simulink model "msm_pi"  (R2021b)
settings: Solver=daessc  StartTime=0.0  StopTime=simlength  MaxStep=Tc  RelTol=1e-3
values from neighbouring files (symbols this model uses):
  A = [-(b+b_theta)/J1 b_theta/J1 -1/J1; b_theta/J2 -(b+b_theta)/J2 1/J2;     k_theta -k_theta 0]    [msm_init.m]
  Ale = [-(b+b_theta)/J1 b_theta/J1 -1/J1 0;         b_theta/J2 -(b+b_theta)/J2 1/J2 1/J2;        k_theta -k_theta 0 0 ... (first row only)    [msm_init.m]
  B = [1/J1 0 0]'    [msm_init.m]
  Ble = [1/J1 0 0 0]'    [msm_init.m]
  C = [1 0 0]    [msm_init.m]
  Cle = [1 0 0 0]    [msm_init.m]
  load_torque = 10    [msm_init.m]
  simlength = 20    [msm_init.m]
  Tc = Ts    (= 0.0001)    [msm_init.m]
undefined symbols (not defined in the file or in its folder): ki1, ki2, kp1, kp2, Ks, L, Lle
libraries: nesl_utility x22, fl_lib x12, mass_spring_mass_lib x4
settings Model: Creator=dbagn  LastModifiedBy=dbagn
settings SolverCC: AlgebraicLoopSolver=TrustRegion
settings DataIOCC: ReturnWorkspaceOutputs=off
settings DebuggingCC: SFMachineParentedDataDiag=warning

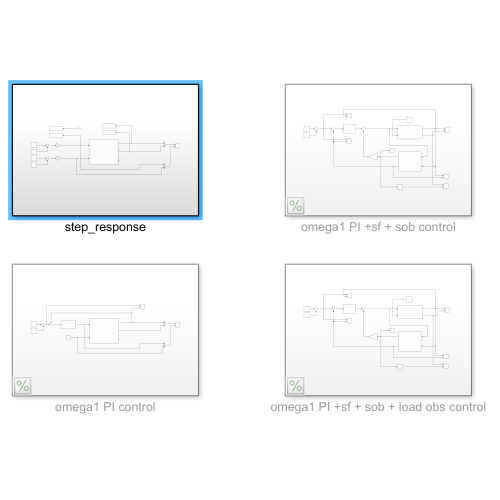
[thumbnail: Simulink's stored preview of the top-level diagram]
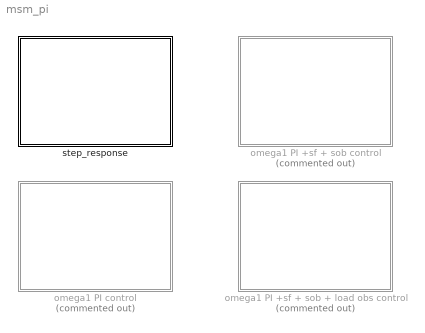
== system msm_pi ==
  omega1 PI +sf + sob + load obs control : Subsystem  Commented=on
  omega1 PI +sf + sob control : Subsystem  Commented=on
  omega1 PI control : Subsystem  Commented=on
  step_response : Subsystem

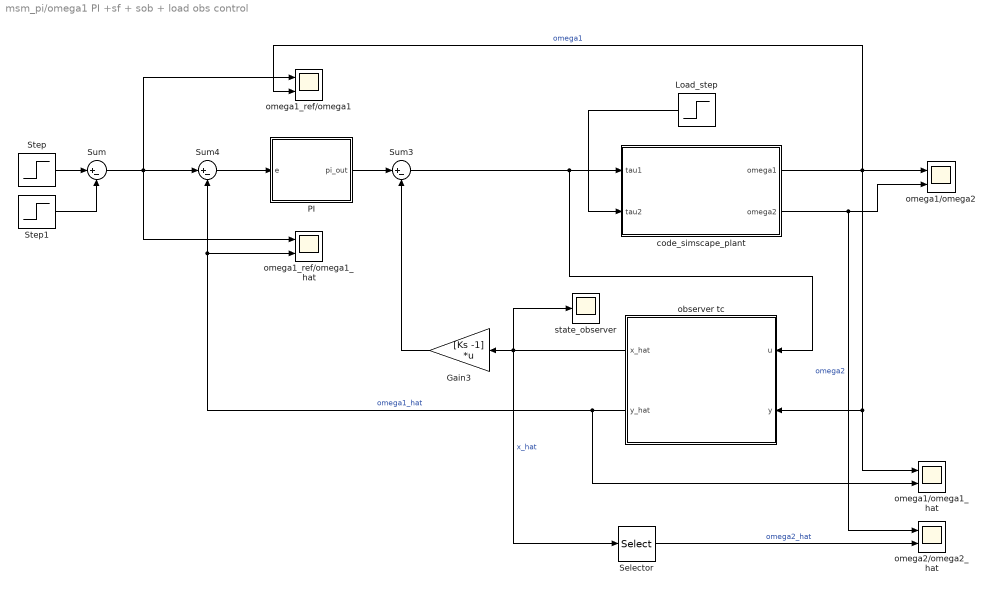
== system msm_pi/omega1 PI +sf + sob + load obs control ==
  Gain3 : Gain  Gain=[Ks -1]  Multiplication=Matrix(K*u)
  Load_step : Step  Time=16  After=load_torque  SampleTime=0
  PI : Subsystem
  Selector : Selector  InputPortWidth=4  IndexOptions=Index vector (dialog)  Indices=2  OutputSizes=1
  Step : Step  Time=0.2  SampleTime=0
  Step1 : Step  Time=8  SampleTime=0
  Sum : Sum  Inputs=|+-
  Sum3 : Sum  Inputs=|+-
  Sum4 : Sum  Inputs=|+-
  "code_simscape_plant " : Subsystem
  observer tc : Subsystem
  omega1/omega1_hat : Scope  NumInputPorts=2
  omega1/omega2 : Scope  NumInputPorts=2
  omega1_ref/omega1 : Scope  NumInputPorts=2
  omega1_ref/omega1_hat : Scope  NumInputPorts=2
  omega2/omega2_hat : Scope  NumInputPorts=2
  state_observer : Scope
  wires:
  PI/1(pi_out) -> Sum3/1
  "code_simscape_plant "/1(omega1) -> observer tc/2(y), omega1/omega1_hat/1, omega1/omega2/1, omega1_ref/omega1/2  "omega1"
  Sum4/1 -> PI/1(e)
  Load_step/1 -> "code_simscape_plant "/2(tau2)
  Gain3/1 -> Sum3/2
  "code_simscape_plant "/2(omega2) -> omega1/omega2/2, omega2/omega2_hat/1  "omega2"
  Selector/1 -> omega2/omega2_hat/2  "omega2_hat"
  observer tc/2(y_hat) -> omega1/omega1_hat/2, Sum4/2, omega1_ref/omega1_hat/2  "omega1_hat"
  observer tc/1(x_hat) -> Gain3/1, state_observer/1, Selector/1  "x_hat"
  Sum3/1 -> observer tc/1(u), "code_simscape_plant "/1(tau1)
  Step1/1 -> Sum/2
  Step/1 -> Sum/1
  Sum/1 -> omega1_ref/omega1_hat/1, Sum4/1, omega1_ref/omega1/1

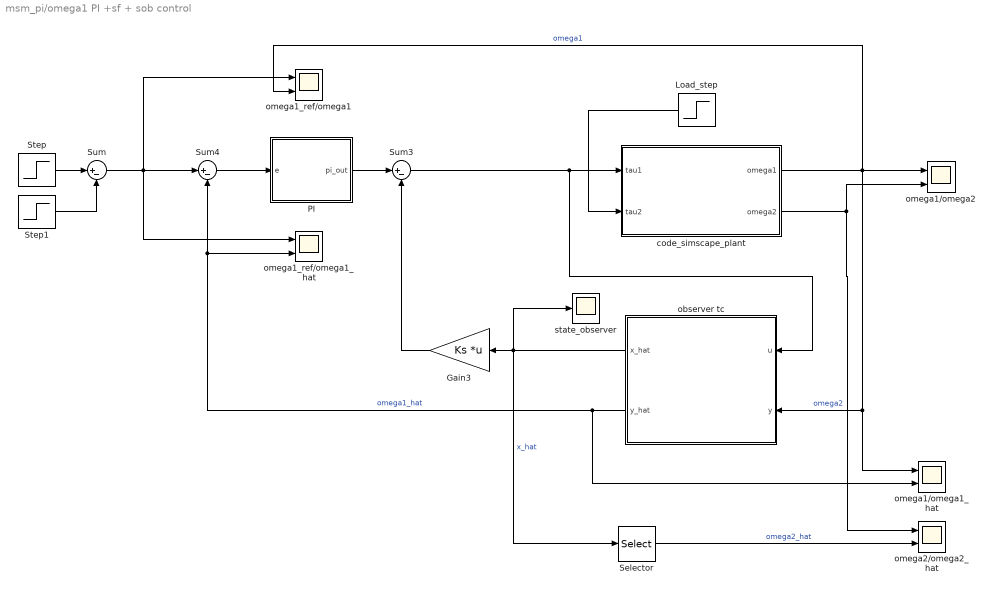
== system msm_pi/omega1 PI +sf + sob control ==
  Gain3 : Gain  Gain=Ks  Multiplication=Matrix(K*u)
  Load_step : Step  Time=16  After=load_torque  SampleTime=0
  PI : Subsystem
  Selector : Selector  InputPortWidth=3  IndexOptions=Index vector (dialog)  Indices=2  OutputSizes=1
  Step : Step  Time=0.2  SampleTime=0
  Step1 : Step  Time=8  SampleTime=0
  Sum : Sum  Inputs=|+-
  Sum3 : Sum  Inputs=|+-
  Sum4 : Sum  Inputs=|+-
  "code_simscape_plant " : Subsystem
  observer tc : Subsystem
  omega1/omega1_hat : Scope  NumInputPorts=2
  omega1/omega2 : Scope  NumInputPorts=2
  omega1_ref/omega1 : Scope  NumInputPorts=2
  omega1_ref/omega1_hat : Scope  NumInputPorts=2
  omega2/omega2_hat : Scope  NumInputPorts=2
  state_observer : Scope
  wires:
  Sum/1 -> omega1_ref/omega1/1, Sum4/1, omega1_ref/omega1_hat/1
  Step/1 -> Sum/1
  Step1/1 -> Sum/2
  Sum3/1 -> "code_simscape_plant "/1(tau1), observer tc/1(u)
  observer tc/1(x_hat) -> Selector/1, state_observer/1, Gain3/1  "x_hat"
  observer tc/2(y_hat) -> omega1_ref/omega1_hat/2, Sum4/2, omega1/omega1_hat/2  "omega1_hat"
  Selector/1 -> omega2/omega2_hat/2  "omega2_hat"
  "code_simscape_plant "/2(omega2) -> omega2/omega2_hat/1, omega1/omega2/2  "omega2"
  Gain3/1 -> Sum3/2
  Load_step/1 -> "code_simscape_plant "/2(tau2)
  Sum4/1 -> PI/1(e)
  "code_simscape_plant "/1(omega1) -> omega1_ref/omega1/2, omega1/omega2/1, omega1/omega1_hat/1, observer tc/2(y)  "omega1"
  PI/1(pi_out) -> Sum3/1

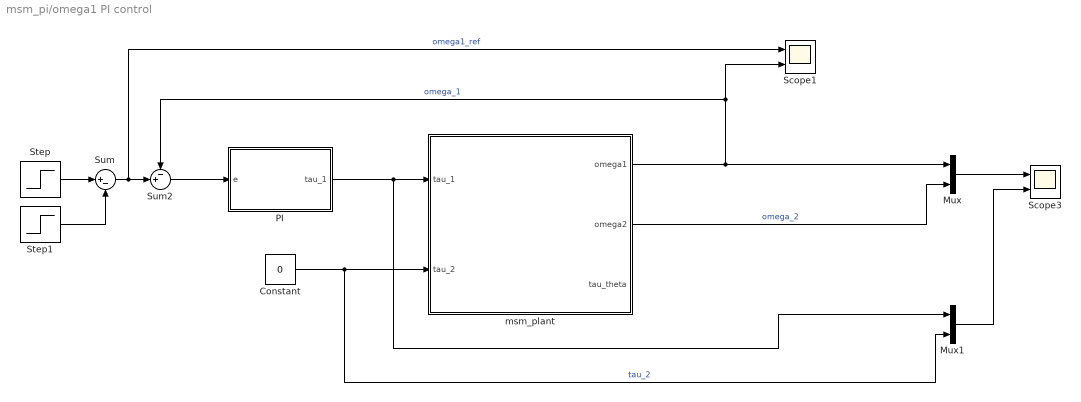
== system msm_pi/omega1 PI control ==
  Constant : Constant  Value=0
  Mux : Mux  Inputs=2
  Mux1 : Mux  Inputs=2
  PI : Subsystem
  Scope1 : Scope  NumInputPorts=2
  Scope3 : Scope  NumInputPorts=2
  Step : Step  Time=0.2  SampleTime=0
  Step1 : Step  Time=simlength/2  SampleTime=0
  Sum : Sum  Inputs=|+-
  Sum2 : Sum  Inputs=-+|
  msm_plant : Subsystem
  wires:
  Mux/1 -> Scope3/1
  Mux1/1 -> Scope3/2
  Step1/1 -> Sum/2
  Step/1 -> Sum/1
  msm_plant/2(omega2) -> Mux/2  "omega_2"
  msm_plant/1(omega1) -> Sum2/1, Scope1/2, Mux/1  "omega_1"
  Constant/1 -> msm_plant/2(tau_2), Mux1/2  "tau_2"
  Sum/1 -> Scope1/1, Sum2/2  "omega1_ref"
  PI/1(tau_1) -> Mux1/1, msm_plant/1(tau_1)
  Sum2/1 -> PI/1(e)

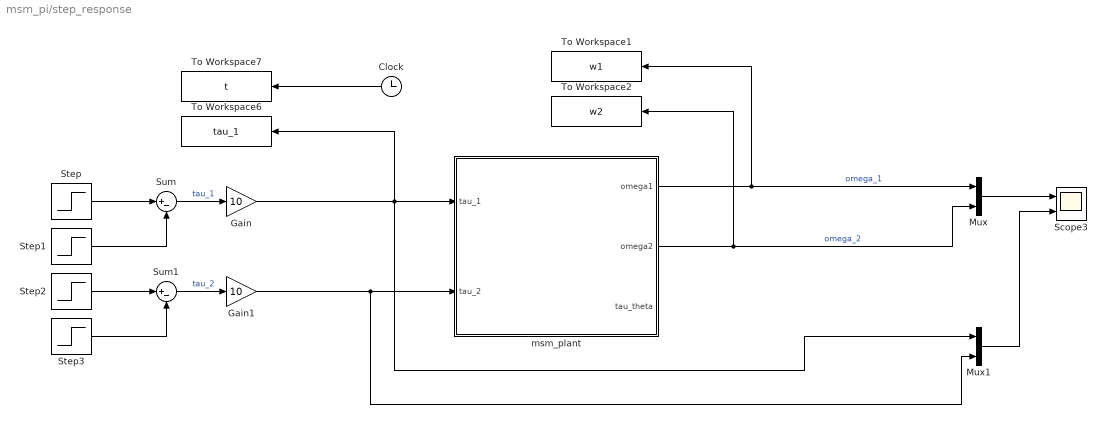
== system msm_pi/step_response ==
  Clock : Clock
  Gain : Gain  Gain=10
  Gain1 : Gain  Gain=10
  Mux : Mux  Inputs=2
  Mux1 : Mux  Inputs=2
  Scope3 : Scope  NumInputPorts=2
  Step : Step  Time=0.2  SampleTime=0
  Step1 : Step  Time=0.25  SampleTime=0
  Step2 : Step  Time=0.2+simlength/2  SampleTime=0
  Step3 : Step  Time=0.25+simlength/2  SampleTime=0
  Sum : Sum  Inputs=|+-
  Sum1 : Sum  Inputs=|+-
  To Workspace1 : ToWorkspace  VariableName=w1  SampleTime=Tc
      settings: MaxDataPoints=Nc
  To Workspace2 : ToWorkspace  VariableName=w2  SampleTime=Tc
      settings: MaxDataPoints=Nc
  To Workspace6 : ToWorkspace  VariableName=tau_1  SampleTime=Tc
      settings: MaxDataPoints=Nc
  To Workspace7 : ToWorkspace  VariableName=t  SampleTime=Tc
      settings: MaxDataPoints=Nc
  msm_plant : Subsystem
  wires:
  Step2/1 -> Sum1/1
  Sum1/1 -> Gain1/1  "tau_2"
  Step3/1 -> Sum1/2
  msm_plant/1(omega1) -> Mux/1, To Workspace1/1  "omega_1"
  Clock/1 -> To Workspace7/1
  msm_plant/2(omega2) -> Mux/2, To Workspace2/1  "omega_2"
  Sum/1 -> Gain/1  "tau_1"
  Step/1 -> Sum/1
  Step1/1 -> Sum/2
  Mux1/1 -> Scope3/2
  Mux/1 -> Scope3/1
  Gain/1 -> To Workspace6/1, Mux1/1, msm_plant/1(tau_1)
  Gain1/1 -> Mux1/2, msm_plant/2(tau_2)

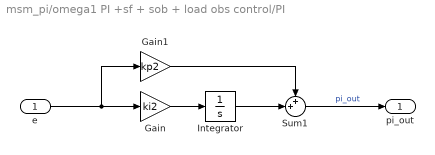
== system msm_pi/omega1 PI +sf + sob + load obs control/PI ==
  e : Inport
  Gain : Gain  Gain=ki2
  Gain1 : Gain  Gain=kp2
  Integrator : Integrator
  Sum1 : Sum  Inputs=++|
  pi_out : Outport
  wires:
  Sum1/1 -> pi_out/1  "pi_out"
  Gain1/1 -> Sum1/1
  Integrator/1 -> Sum1/2
  Gain/1 -> Integrator/1
  e/1 -> Gain1/1, Gain/1

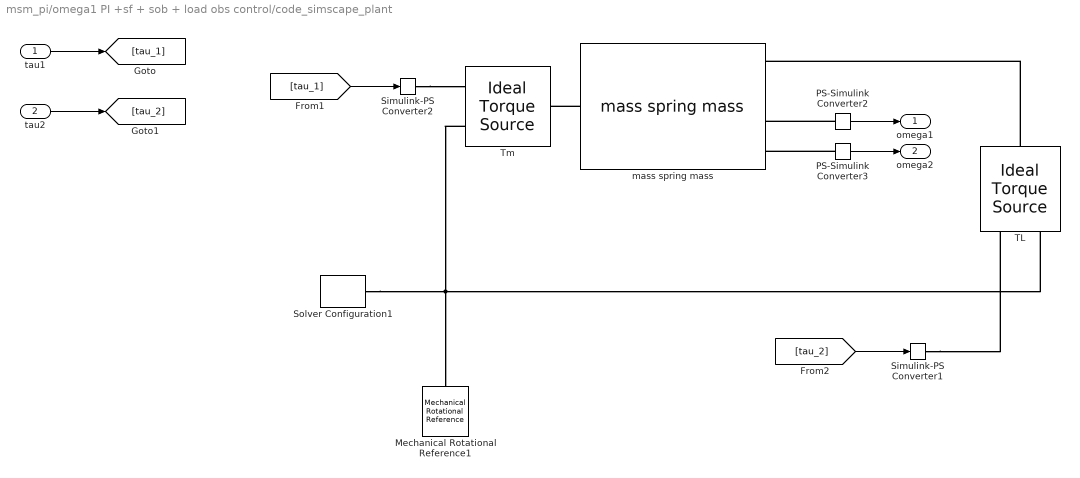
== system msm_pi/omega1 PI +sf + sob + load obs control/code_simscape_plant  ==
  tau1 : Inport
  tau2 : Inport  Port=2
  Mechanical Rotational Reference1 : fl_lib/Mechanical/Rotational Elements/Mechanical Rotational Reference
  PS-Simulink Converter2 : nesl_utility/PS-Simulink Converter  PhysicalDomain=network_engine_domain  SubClassName=ps_output  LeftPortType=input  RightPortType=output  PseudoPeriodic=off  Frequencies=[]  Unit=1  AffineConversion=off
      settings: SourceProductBaseCode=PW,SS
  PS-Simulink Converter3 : nesl_utility/PS-Simulink Converter  PhysicalDomain=network_engine_domain  SubClassName=ps_output  LeftPortType=input  RightPortType=output  PseudoPeriodic=off  Frequencies=[]  Unit=1  AffineConversion=off
      settings: SourceProductBaseCode=PW,SS
  Simulink-PS Converter1 : nesl_utility/Simulink-PS Converter  PhysicalDomain=network_engine_domain  SubClassName=ps_input  LeftPortType=input  RightPortType=output  PseudoPeriodic=off  Frequencies=[]  NoiseDistribution=none  NoiseParameters=[]  Unit=1  AffineConversion=off  FilteringAndDerivatives=provide  SimscapeFilterOrder=1  InputFilterTimeConstant=0.001  UdotUserProvided=0
      settings: SourceProductBaseCode=PW,SS
  Simulink-PS Converter2 : nesl_utility/Simulink-PS Converter  PhysicalDomain=network_engine_domain  SubClassName=ps_input  LeftPortType=input  RightPortType=output  PseudoPeriodic=off  Frequencies=[]  NoiseDistribution=none  NoiseParameters=[]  Unit=1  AffineConversion=off  FilteringAndDerivatives=provide  SimscapeFilterOrder=1  InputFilterTimeConstant=0.001  UdotUserProvided=0
      settings: SourceProductBaseCode=PW,SS
  Solver Configuration1 : nesl_utility/Solver Configuration  PhysicalDomain=network_engine_domain  SubClassName=solver  LeftPortType=input  RightPortType=generic  Tones=[]  Harmonics=[]  SimulateNoise=off  Profile=off  UseLocalSampling=off  EnableSwitchedLinearOptims=on  FrequencyDomain=off  UseCCode=off  RelTol=0.001  AbsTol=1e-06  MinStep=1e-09  ToWorkspace=off  RevertToSquareIcSolve=off  NumHomotopyIterations=100  PhasorMode=off  PhasorModeNumHarmonics=1  DoDC=off  ResidualTolerance=1e-09  UseLocalSolver=off  LocalSolverChoice=NE_BACKWARD_EULER_ADVANCER  LocalSolverSampleTime=0.001  DoFixedCost=off  MaxNonlinIter=3  MaxModeIter=2  ComputeImpulses=off  ImpulseIterations=2  LinearAlgebra=auto  EquationFormulation=NE_TIME_EF  DelaysMemoryBudget=1024  AutomaticFiltering=on  FilteringTimeConstant=0.001  PartitionStorageMethod=AS_NEEDED  PartitionMemoryBudget=1024  PartitionMethod=ROBUST
      settings: SourceProductBaseCode=PW,SS
  TL : fl_lib/Mechanical/Mechanical Sources/Ideal Torque Source
  "Tm " : fl_lib/Mechanical/Mechanical Sources/Ideal Torque Source
  mass spring mass : mass_spring_mass_lib/mass spring mass  b1=b N*m/(rad/s)  J1=J1 kg*m^2  b2=b N*m/(rad/s)  J2=J2 kg*m^2  b_theta=b_theta N*m/(rad/s)  k_theta=k_theta N*m/rad  omega_1_specify=off  omega_1_priority=None  omega_1=0 rad/s  omega_1_nominal_specify=off  omega_1_nominal_unit=rad/s  omega_1_nominal_value=1  omega_2_specify=off  omega_2_priority=None  omega_2=0 rad/s  omega_2_nominal_specify=off  omega_2_nominal_unit=rad/s  omega_2_nominal_value=1  tau_1_specify=off  tau_1_priority=None  tau_1=0 N*m  tau_1_nominal_specify=off  tau_1_nominal_unit=N*m  tau_1_nominal_value=1  tau_2_specify=off  tau_2_priority=None  tau_2=0 N*m  tau_2_nominal_specify=off  tau_2_nominal_unit=N*m  tau_2_nominal_value=1  tau_theta_specify=off  tau_theta_priority=None  tau_theta=0 N*m  tau_theta_nominal_specify=off  tau_theta_nominal_unit=N*m  tau_theta_nominal_value=1
      settings: InternalSimscapePortConfiguration="{\"Bottom\":[],\"Left\":[{\"id\":\"S1\",\"label\":\"S1\",\"type\":\"foundation.mechanical.rotational.rotational\"}],\"Right\":[{\"id\":\"S2\",\"label\":\"S2\",\"type\":\"foundation.mechanical.rotational.rotational\"},{\"id\":\"tau_theta_out\",\"label\":\"tau_theta\",\"type\":\"output\"},{\"id\":\"omega1_out\",\"label\":\"omega1\",\"type\":\"output\"},{\"id\":\"omega2_out\",\"label\":\"omega2\",\"type\":\"output\"}],\"Top\":[]}"
  omega1 : Outport
  omega2 : Outport  Port=2
  wires:
  PS-Simulink Converter2/1 -> omega1/1
  PS-Simulink Converter3/1 -> omega2/1
  tau1/1 -> [tau_1]
  [tau_1] -> Simulink-PS Converter2/1
  tau2/1 -> [tau_2]
  [tau_2] -> Simulink-PS Converter1/1
  connections:
  TL/RConn2 -- Mechanical Rotational Reference1/LConn1 -- "Tm "/RConn2 -- Solver Configuration1/RConn1
  PS-Simulink Converter2/LConn1 -- mass spring mass/RConn3
  PS-Simulink Converter3/LConn1 -- mass spring mass/RConn4
  TL/LConn1 -- mass spring mass/RConn1
  Simulink-PS Converter1/RConn1 -- TL/RConn1
  mass spring mass/LConn1 -- "Tm "/LConn1
  Simulink-PS Converter2/RConn1 -- "Tm "/RConn1

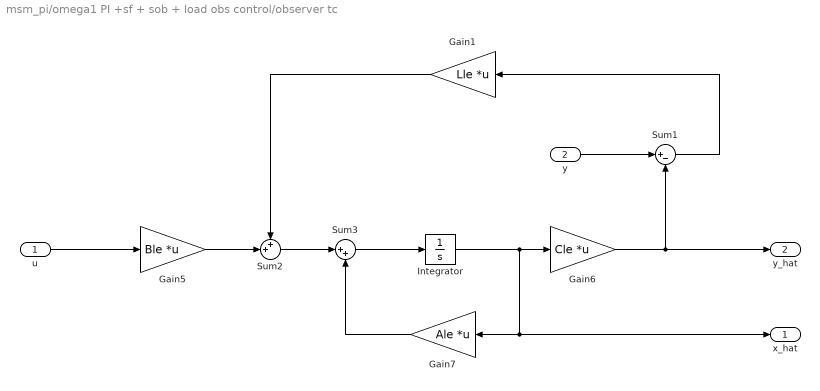
== system msm_pi/omega1 PI +sf + sob + load obs control/observer tc ==
  u : Inport
  y : Inport  Port=2
  Gain1 : Gain  Gain=Lle  Multiplication=Matrix(K*u)
  Gain5 : Gain  Gain=Ble  Multiplication=Matrix(K*u)
  Gain6 : Gain  Gain=Cle  Multiplication=Matrix(K*u)
  Gain7 : Gain  Gain=Ale  Multiplication=Matrix(K*u)
  Integrator : Integrator
  Sum1 : Sum  Inputs=|+-
  Sum2 : Sum  Inputs=++|
  Sum3 : Sum  Inputs=|++
  x_hat : Outport
  y_hat : Outport  Port=2
  wires:
  Gain5/1 -> Sum2/2
  Gain1/1 -> Sum2/1
  u/1 -> Gain5/1
  Sum1/1 -> Gain1/1
  Gain6/1 -> Sum1/2, y_hat/1
  y/1 -> Sum1/1
  Gain7/1 -> Sum3/2
  Sum2/1 -> Sum3/1
  Sum3/1 -> Integrator/1
  Integrator/1 -> Gain6/1, Gain7/1, x_hat/1

== system msm_pi/omega1 PI +sf + sob control/PI ==
  e : Inport
  Gain : Gain  Gain=ki2
  Gain1 : Gain  Gain=kp2
  Integrator : Integrator
  Sum1 : Sum  Inputs=++|
  pi_out : Outport
  wires:
  e/1 -> Gain/1, Gain1/1
  Gain/1 -> Integrator/1
  Integrator/1 -> Sum1/2
  Gain1/1 -> Sum1/1
  Sum1/1 -> pi_out/1  "pi_out"

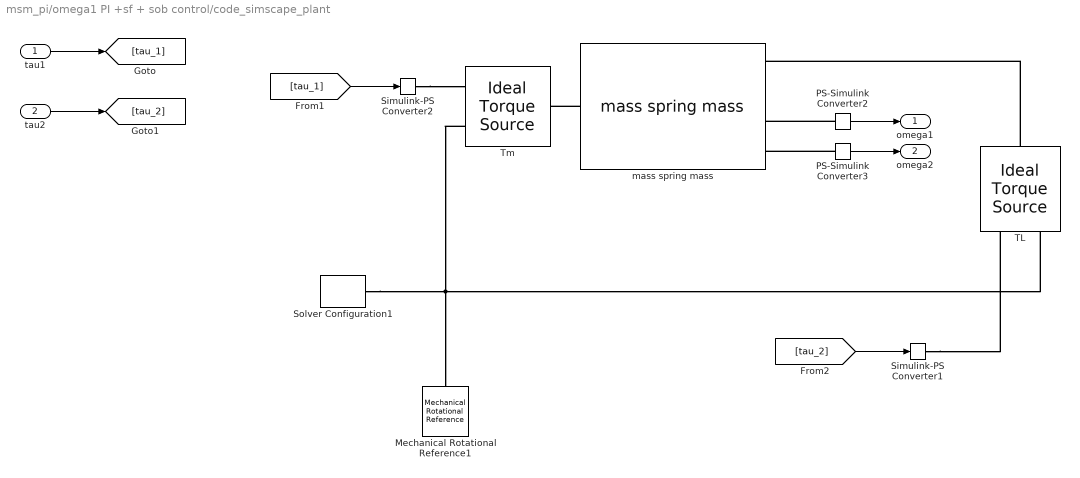
== system msm_pi/omega1 PI +sf + sob control/code_simscape_plant  ==
  tau1 : Inport
  tau2 : Inport  Port=2
  Mechanical Rotational Reference1 : fl_lib/Mechanical/Rotational Elements/Mechanical Rotational Reference
  PS-Simulink Converter2 : nesl_utility/PS-Simulink Converter  PhysicalDomain=network_engine_domain  SubClassName=ps_output  LeftPortType=input  RightPortType=output  PseudoPeriodic=off  Frequencies=[]  Unit=1  AffineConversion=off
      settings: SourceProductBaseCode=PW,SS
  PS-Simulink Converter3 : nesl_utility/PS-Simulink Converter  PhysicalDomain=network_engine_domain  SubClassName=ps_output  LeftPortType=input  RightPortType=output  PseudoPeriodic=off  Frequencies=[]  Unit=1  AffineConversion=off
      settings: SourceProductBaseCode=PW,SS
  Simulink-PS Converter1 : nesl_utility/Simulink-PS Converter  PhysicalDomain=network_engine_domain  SubClassName=ps_input  LeftPortType=input  RightPortType=output  PseudoPeriodic=off  Frequencies=[]  NoiseDistribution=none  NoiseParameters=[]  Unit=1  AffineConversion=off  FilteringAndDerivatives=provide  SimscapeFilterOrder=1  InputFilterTimeConstant=0.001  UdotUserProvided=0
      settings: SourceProductBaseCode=PW,SS
  Simulink-PS Converter2 : nesl_utility/Simulink-PS Converter  PhysicalDomain=network_engine_domain  SubClassName=ps_input  LeftPortType=input  RightPortType=output  PseudoPeriodic=off  Frequencies=[]  NoiseDistribution=none  NoiseParameters=[]  Unit=1  AffineConversion=off  FilteringAndDerivatives=provide  SimscapeFilterOrder=1  InputFilterTimeConstant=0.001  UdotUserProvided=0
      settings: SourceProductBaseCode=PW,SS
  Solver Configuration1 : nesl_utility/Solver Configuration  PhysicalDomain=network_engine_domain  SubClassName=solver  LeftPortType=input  RightPortType=generic  Tones=[]  Harmonics=[]  SimulateNoise=off  Profile=off  UseLocalSampling=off  EnableSwitchedLinearOptims=on  FrequencyDomain=off  UseCCode=off  RelTol=0.001  AbsTol=1e-06  MinStep=1e-09  ToWorkspace=off  RevertToSquareIcSolve=off  NumHomotopyIterations=100  PhasorMode=off  PhasorModeNumHarmonics=1  DoDC=off  ResidualTolerance=1e-09  UseLocalSolver=off  LocalSolverChoice=NE_BACKWARD_EULER_ADVANCER  LocalSolverSampleTime=0.001  DoFixedCost=off  MaxNonlinIter=3  MaxModeIter=2  ComputeImpulses=off  ImpulseIterations=2  LinearAlgebra=auto  EquationFormulation=NE_TIME_EF  DelaysMemoryBudget=1024  AutomaticFiltering=on  FilteringTimeConstant=0.001  PartitionStorageMethod=AS_NEEDED  PartitionMemoryBudget=1024  PartitionMethod=ROBUST
      settings: SourceProductBaseCode=PW,SS
  TL : fl_lib/Mechanical/Mechanical Sources/Ideal Torque Source
  "Tm " : fl_lib/Mechanical/Mechanical Sources/Ideal Torque Source
  mass spring mass : mass_spring_mass_lib/mass spring mass  b1=b N*m/(rad/s)  J1=J1 kg*m^2  b2=b N*m/(rad/s)  J2=J2 kg*m^2  b_theta=b_theta N*m/(rad/s)  k_theta=k_theta N*m/rad  omega_1_specify=off  omega_1_priority=None  omega_1=0 rad/s  omega_1_nominal_specify=off  omega_1_nominal_unit=rad/s  omega_1_nominal_value=1  omega_2_specify=off  omega_2_priority=None  omega_2=0 rad/s  omega_2_nominal_specify=off  omega_2_nominal_unit=rad/s  omega_2_nominal_value=1  tau_1_specify=off  tau_1_priority=None  tau_1=0 N*m  tau_1_nominal_specify=off  tau_1_nominal_unit=N*m  tau_1_nominal_value=1  tau_2_specify=off  tau_2_priority=None  tau_2=0 N*m  tau_2_nominal_specify=off  tau_2_nominal_unit=N*m  tau_2_nominal_value=1  tau_theta_specify=off  tau_theta_priority=None  tau_theta=0 N*m  tau_theta_nominal_specify=off  tau_theta_nominal_unit=N*m  tau_theta_nominal_value=1
      settings: InternalSimscapePortConfiguration="{\"Bottom\":[],\"Left\":[{\"id\":\"S1\",\"label\":\"S1\",\"type\":\"foundation.mechanical.rotational.rotational\"}],\"Right\":[{\"id\":\"S2\",\"label\":\"S2\",\"type\":\"foundation.mechanical.rotational.rotational\"},{\"id\":\"tau_theta_out\",\"label\":\"tau_theta\",\"type\":\"output\"},{\"id\":\"omega1_out\",\"label\":\"omega1\",\"type\":\"output\"},{\"id\":\"omega2_out\",\"label\":\"omega2\",\"type\":\"output\"}],\"Top\":[]}"
  omega1 : Outport
  omega2 : Outport  Port=2
  wires:
  [tau_2] -> Simulink-PS Converter1/1
  tau2/1 -> [tau_2]
  [tau_1] -> Simulink-PS Converter2/1
  tau1/1 -> [tau_1]
  PS-Simulink Converter3/1 -> omega2/1
  PS-Simulink Converter2/1 -> omega1/1
  connections:
  Simulink-PS Converter2/RConn1 -- "Tm "/RConn1
  mass spring mass/LConn1 -- "Tm "/LConn1
  Simulink-PS Converter1/RConn1 -- TL/RConn1
  TL/LConn1 -- mass spring mass/RConn1
  PS-Simulink Converter3/LConn1 -- mass spring mass/RConn4
  PS-Simulink Converter2/LConn1 -- mass spring mass/RConn3
  Solver Configuration1/RConn1 -- "Tm "/RConn2 -- Mechanical Rotational Reference1/LConn1 -- TL/RConn2

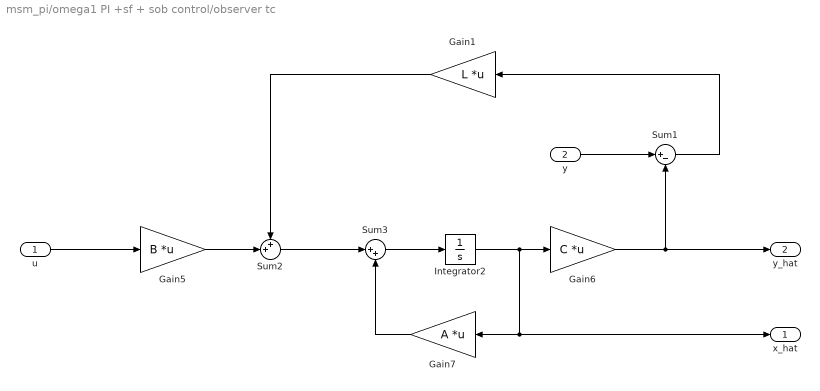
== system msm_pi/omega1 PI +sf + sob control/observer tc ==
  u : Inport
  y : Inport  Port=2
  Gain1 : Gain  Gain=L  Multiplication=Matrix(K*u)
  Gain5 : Gain  Gain=B  Multiplication=Matrix(K*u)
  Gain6 : Gain  Gain=C  Multiplication=Matrix(K*u)
  Gain7 : Gain  Gain=A  Multiplication=Matrix(K*u)
  Integrator2 : Integrator
  Sum1 : Sum  Inputs=|+-
  Sum2 : Sum  Inputs=++|
  Sum3 : Sum  Inputs=|++
  x_hat : Outport
  y_hat : Outport  Port=2
  wires:
  Sum2/1 -> Sum3/1
  Integrator2/1 -> x_hat/1, Gain7/1, Gain6/1
  Sum3/1 -> Integrator2/1
  Gain7/1 -> Sum3/2
  y/1 -> Sum1/1
  Gain6/1 -> y_hat/1, Sum1/2
  Sum1/1 -> Gain1/1
  u/1 -> Gain5/1
  Gain1/1 -> Sum2/1
  Gain5/1 -> Sum2/2

== system msm_pi/omega1 PI control/PI ==
  e : Inport
  Gain : Gain  Gain=ki1
  Gain1 : Gain  Gain=kp1
  Integrator : Integrator
  Sum1 : Sum  Inputs=++|
  tau_1 : Outport
  wires:
  Sum1/1 -> tau_1/1  "tau_1"
  Gain/1 -> Integrator/1
  Gain1/1 -> Sum1/1
  Integrator/1 -> Sum1/2
  e/1 -> Gain1/1, Gain/1

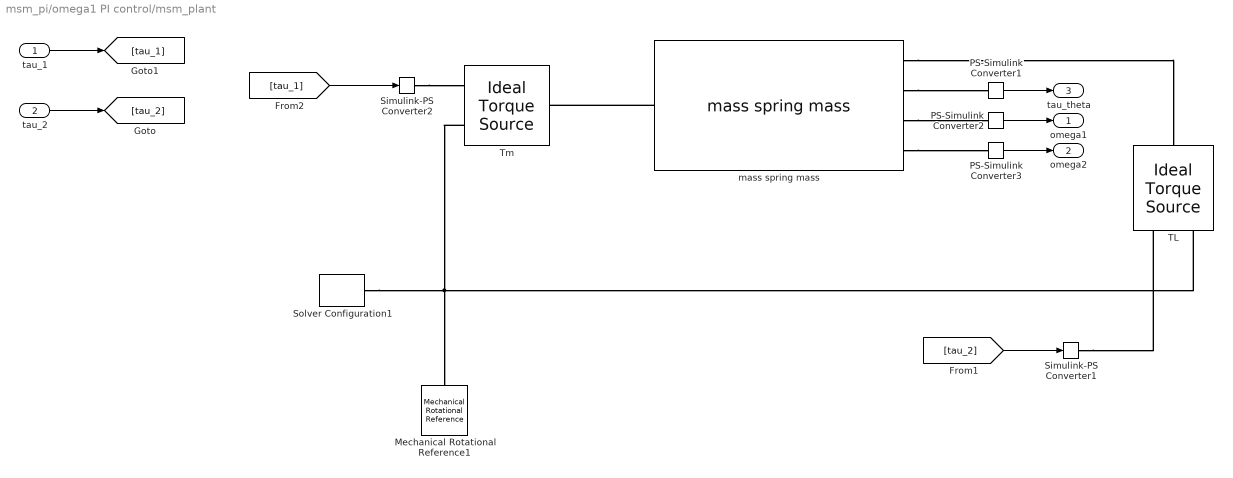
== system msm_pi/omega1 PI control/msm_plant ==
  tau_1 : Inport
  tau_2 : Inport  Port=2
  Mechanical Rotational Reference1 : fl_lib/Mechanical/Rotational Elements/Mechanical Rotational Reference
  PS-Simulink Converter1 : nesl_utility/PS-Simulink Converter  PhysicalDomain=network_engine_domain  SubClassName=ps_output  LeftPortType=input  RightPortType=output  PseudoPeriodic=off  Frequencies=[]  Unit=1  AffineConversion=off
      settings: SourceProductBaseCode=PW,SS
  PS-Simulink Converter2 : nesl_utility/PS-Simulink Converter  PhysicalDomain=network_engine_domain  SubClassName=ps_output  LeftPortType=input  RightPortType=output  PseudoPeriodic=off  Frequencies=[]  Unit=1  AffineConversion=off
      settings: SourceProductBaseCode=PW,SS
  PS-Simulink Converter3 : nesl_utility/PS-Simulink Converter  PhysicalDomain=network_engine_domain  SubClassName=ps_output  LeftPortType=input  RightPortType=output  PseudoPeriodic=off  Frequencies=[]  Unit=1  AffineConversion=off
      settings: SourceProductBaseCode=PW,SS
  Simulink-PS Converter1 : nesl_utility/Simulink-PS Converter  PhysicalDomain=network_engine_domain  SubClassName=ps_input  LeftPortType=input  RightPortType=output  PseudoPeriodic=off  Frequencies=[]  NoiseDistribution=none  NoiseParameters=[]  Unit=1  AffineConversion=off  FilteringAndDerivatives=provide  SimscapeFilterOrder=1  InputFilterTimeConstant=0.001  UdotUserProvided=0
      settings: SourceProductBaseCode=PW,SS
  Simulink-PS Converter2 : nesl_utility/Simulink-PS Converter  PhysicalDomain=network_engine_domain  SubClassName=ps_input  LeftPortType=input  RightPortType=output  PseudoPeriodic=off  Frequencies=[]  NoiseDistribution=none  NoiseParameters=[]  Unit=1  AffineConversion=off  FilteringAndDerivatives=provide  SimscapeFilterOrder=1  InputFilterTimeConstant=0.001  UdotUserProvided=0
      settings: SourceProductBaseCode=PW,SS
  Solver Configuration1 : nesl_utility/Solver Configuration  PhysicalDomain=network_engine_domain  SubClassName=solver  LeftPortType=input  RightPortType=generic  Tones=[]  Harmonics=[]  SimulateNoise=off  Profile=off  UseLocalSampling=off  EnableSwitchedLinearOptims=on  FrequencyDomain=off  UseCCode=off  RelTol=0.001  AbsTol=1e-06  MinStep=1e-09  ToWorkspace=off  RevertToSquareIcSolve=off  NumHomotopyIterations=100  PhasorMode=off  PhasorModeNumHarmonics=1  DoDC=off  ResidualTolerance=1e-09  UseLocalSolver=off  LocalSolverChoice=NE_BACKWARD_EULER_ADVANCER  LocalSolverSampleTime=Ts  DoFixedCost=off  MaxNonlinIter=3  MaxModeIter=2  ComputeImpulses=off  ImpulseIterations=2  LinearAlgebra=auto  EquationFormulation=NE_TIME_EF  DelaysMemoryBudget=1024  AutomaticFiltering=on  FilteringTimeConstant=0.001  PartitionStorageMethod=AS_NEEDED  PartitionMemoryBudget=1024  PartitionMethod=ROBUST
      settings: SourceProductBaseCode=PW,SS
  TL : fl_lib/Mechanical/Mechanical Sources/Ideal Torque Source
  "Tm " : fl_lib/Mechanical/Mechanical Sources/Ideal Torque Source
  mass spring mass : mass_spring_mass_lib/mass spring mass  b1=b N*m/(rad/s)  J1=J1 kg*m^2  b2=b N*m/(rad/s)  J2=J2 kg*m^2  b_theta=b_theta N*m/(rad/s)  k_theta=k_theta N*m/rad  omega_1_specify=off  omega_1_priority=None  omega_1=0 rad/s  omega_1_nominal_specify=off  omega_1_nominal_unit=rad/s  omega_1_nominal_value=1  omega_2_specify=off  omega_2_priority=None  omega_2=0 rad/s  omega_2_nominal_specify=off  omega_2_nominal_unit=rad/s  omega_2_nominal_value=1  tau_1_specify=off  tau_1_priority=None  tau_1=0 N*m  tau_1_nominal_specify=off  tau_1_nominal_unit=N*m  tau_1_nominal_value=1  tau_2_specify=off  tau_2_priority=None  tau_2=0 N*m  tau_2_nominal_specify=off  tau_2_nominal_unit=N*m  tau_2_nominal_value=1  tau_theta_specify=off  tau_theta_priority=None  tau_theta=0 N*m  tau_theta_nominal_specify=off  tau_theta_nominal_unit=N*m  tau_theta_nominal_value=1
      settings: InternalSimscapePortConfiguration="{\"Bottom\":[],\"Left\":[{\"id\":\"S1\",\"label\":\"S1\",\"type\":\"foundation.mechanical.rotational.rotational\"}],\"Right\":[{\"id\":\"S2\",\"label\":\"S2\",\"type\":\"foundation.mechanical.rotational.rotational\"},{\"id\":\"tau_theta_out\",\"label\":\"tau_theta\",\"type\":\"output\"},{\"id\":\"omega1_out\",\"label\":\"omega1\",\"type\":\"output\"},{\"id\":\"omega2_out\",\"label\":\"omega2\",\"type\":\"output\"}],\"Top\":[]}"
  omega1 : Outport
  omega2 : Outport  Port=2
  tau_theta : Outport  Port=3
  wires:
  PS-Simulink Converter1/1 -> tau_theta/1
  [tau_2] -> Simulink-PS Converter1/1
  [tau_1] -> Simulink-PS Converter2/1
  tau_2/1 -> [tau_2]
  tau_1/1 -> [tau_1]
  PS-Simulink Converter2/1 -> omega1/1
  PS-Simulink Converter3/1 -> omega2/1
  connections:
  mass spring mass/RConn2 -- PS-Simulink Converter1/LConn1
  TL/RConn2 -- Mechanical Rotational Reference1/LConn1 -- "Tm "/RConn2 -- Solver Configuration1/RConn1
  mass spring mass/RConn3 -- PS-Simulink Converter2/LConn1
  mass spring mass/RConn4 -- PS-Simulink Converter3/LConn1
  mass spring mass/RConn1 -- TL/LConn1
  Simulink-PS Converter1/RConn1 -- TL/RConn1
  mass spring mass/LConn1 -- "Tm "/LConn1
  Simulink-PS Converter2/RConn1 -- "Tm "/RConn1

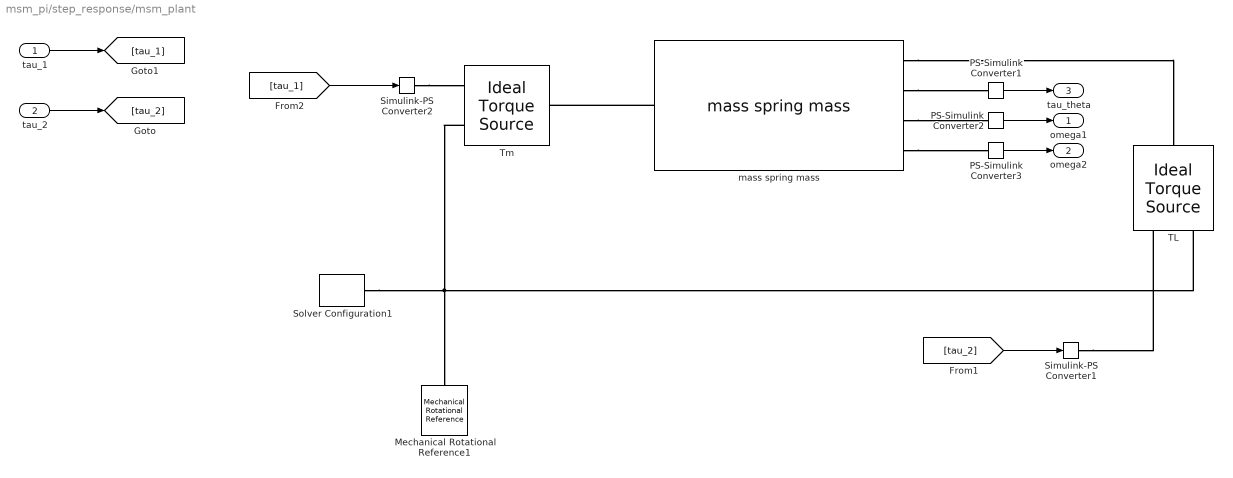
== system msm_pi/step_response/msm_plant ==
  tau_1 : Inport
  tau_2 : Inport  Port=2
  Mechanical Rotational Reference1 : fl_lib/Mechanical/Rotational Elements/Mechanical Rotational Reference
  PS-Simulink Converter1 : nesl_utility/PS-Simulink Converter  PhysicalDomain=network_engine_domain  SubClassName=ps_output  LeftPortType=input  RightPortType=output  PseudoPeriodic=off  Frequencies=[]  Unit=1  AffineConversion=off
      settings: SourceProductBaseCode=PW,SS
  PS-Simulink Converter2 : nesl_utility/PS-Simulink Converter  PhysicalDomain=network_engine_domain  SubClassName=ps_output  LeftPortType=input  RightPortType=output  PseudoPeriodic=off  Frequencies=[]  Unit=1  AffineConversion=off
      settings: SourceProductBaseCode=PW,SS
  PS-Simulink Converter3 : nesl_utility/PS-Simulink Converter  PhysicalDomain=network_engine_domain  SubClassName=ps_output  LeftPortType=input  RightPortType=output  PseudoPeriodic=off  Frequencies=[]  Unit=1  AffineConversion=off
      settings: SourceProductBaseCode=PW,SS
  Simulink-PS Converter1 : nesl_utility/Simulink-PS Converter  PhysicalDomain=network_engine_domain  SubClassName=ps_input  LeftPortType=input  RightPortType=output  PseudoPeriodic=off  Frequencies=[]  NoiseDistribution=none  NoiseParameters=[]  Unit=1  AffineConversion=off  FilteringAndDerivatives=provide  SimscapeFilterOrder=1  InputFilterTimeConstant=0.001  UdotUserProvided=0
      settings: SourceProductBaseCode=PW,SS
  Simulink-PS Converter2 : nesl_utility/Simulink-PS Converter  PhysicalDomain=network_engine_domain  SubClassName=ps_input  LeftPortType=input  RightPortType=output  PseudoPeriodic=off  Frequencies=[]  NoiseDistribution=none  NoiseParameters=[]  Unit=1  AffineConversion=off  FilteringAndDerivatives=provide  SimscapeFilterOrder=1  InputFilterTimeConstant=0.001  UdotUserProvided=0
      settings: SourceProductBaseCode=PW,SS
  Solver Configuration1 : nesl_utility/Solver Configuration  PhysicalDomain=network_engine_domain  SubClassName=solver  LeftPortType=input  RightPortType=generic  Tones=[]  Harmonics=[]  SimulateNoise=off  Profile=off  UseLocalSampling=off  EnableSwitchedLinearOptims=on  FrequencyDomain=off  UseCCode=off  RelTol=0.001  AbsTol=1e-06  MinStep=1e-09  ToWorkspace=off  RevertToSquareIcSolve=off  NumHomotopyIterations=100  PhasorMode=off  PhasorModeNumHarmonics=1  DoDC=off  ResidualTolerance=1e-09  UseLocalSolver=off  LocalSolverChoice=NE_BACKWARD_EULER_ADVANCER  LocalSolverSampleTime=0.001  DoFixedCost=off  MaxNonlinIter=3  MaxModeIter=2  ComputeImpulses=off  ImpulseIterations=2  LinearAlgebra=auto  EquationFormulation=NE_TIME_EF  DelaysMemoryBudget=1024  AutomaticFiltering=on  FilteringTimeConstant=0.001  PartitionStorageMethod=AS_NEEDED  PartitionMemoryBudget=1024  PartitionMethod=ROBUST
      settings: SourceProductBaseCode=PW,SS
  TL : fl_lib/Mechanical/Mechanical Sources/Ideal Torque Source
  "Tm " : fl_lib/Mechanical/Mechanical Sources/Ideal Torque Source
  mass spring mass : mass_spring_mass_lib/mass spring mass  b1=b N*m/(rad/s)  J1=J1 kg*m^2  b2=b N*m/(rad/s)  J2=J2 kg*m^2  b_theta=b_theta N*m/(rad/s)  k_theta=k_theta N*m/rad  omega_1_specify=off  omega_1_priority=None  omega_1=0 rad/s  omega_1_nominal_specify=off  omega_1_nominal_unit=rad/s  omega_1_nominal_value=1  omega_2_specify=off  omega_2_priority=None  omega_2=0 rad/s  omega_2_nominal_specify=off  omega_2_nominal_unit=rad/s  omega_2_nominal_value=1  tau_1_specify=off  tau_1_priority=None  tau_1=0 N*m  tau_1_nominal_specify=off  tau_1_nominal_unit=N*m  tau_1_nominal_value=1  tau_2_specify=off  tau_2_priority=None  tau_2=0 N*m  tau_2_nominal_specify=off  tau_2_nominal_unit=N*m  tau_2_nominal_value=1  tau_theta_specify=off  tau_theta_priority=None  tau_theta=0 N*m  tau_theta_nominal_specify=off  tau_theta_nominal_unit=N*m  tau_theta_nominal_value=1
      settings: InternalSimscapePortConfiguration="{\"Bottom\":[],\"Left\":[{\"id\":\"S1\",\"label\":\"S1\",\"type\":\"foundation.mechanical.rotational.rotational\"}],\"Right\":[{\"id\":\"S2\",\"label\":\"S2\",\"type\":\"foundation.mechanical.rotational.rotational\"},{\"id\":\"tau_theta_out\",\"label\":\"tau_theta\",\"type\":\"output\"},{\"id\":\"omega1_out\",\"label\":\"omega1\",\"type\":\"output\"},{\"id\":\"omega2_out\",\"label\":\"omega2\",\"type\":\"output\"}],\"Top\":[]}"
  omega1 : Outport
  omega2 : Outport  Port=2
  tau_theta : Outport  Port=3
  wires:
  PS-Simulink Converter3/1 -> omega2/1
  PS-Simulink Converter2/1 -> omega1/1
  tau_1/1 -> [tau_1]
  tau_2/1 -> [tau_2]
  [tau_1] -> Simulink-PS Converter2/1
  [tau_2] -> Simulink-PS Converter1/1
  PS-Simulink Converter1/1 -> tau_theta/1
  connections:
  Simulink-PS Converter2/RConn1 -- "Tm "/RConn1
  mass spring mass/LConn1 -- "Tm "/LConn1
  Simulink-PS Converter1/RConn1 -- TL/RConn1
  mass spring mass/RConn1 -- TL/LConn1
  mass spring mass/RConn4 -- PS-Simulink Converter3/LConn1
  mass spring mass/RConn3 -- PS-Simulink Converter2/LConn1
  Solver Configuration1/RConn1 -- "Tm "/RConn2 -- Mechanical Rotational Reference1/LConn1 -- TL/RConn2
  mass spring mass/RConn2 -- PS-Simulink Converter1/LConn1
